simulink model "Controladores_valvula"  (R2014a)
settings: Solver=ode45  StartTime=0.0  StopTime=60  MaxStep=0.1  RelTol=1e-3
values from neighbouring files (symbols this model uses):
  Ap0 = 49.978    [Seccion_5.m]
  Fh0 = 0.8946    [Seccion_5.m]
  Kc_CC_v = 180.7564    [Seccion_5.m]
  Kc_IMC_v = 111.7318    [Seccion_5.m]
  Kc_ZN_v = 155.1600    (= 155.16)    [Seccion_5.m]
  KcPIM_IMC_v = 127.6824    [Seccion_5.m]
  Ki_CC_v = Kc_CC_v/Taoi_CC_v    (= 86.2346262106)    [Seccion_5.m]
  Ki_IMC_v = Kc_IMC_v/Taoi_IMC_v    (= 31.9233714286)    [Seccion_5.m]
  Ki_ZN_v = Kc_ZN_v/Taoi_ZN_v    (= 51.5704457074)    [Seccion_5.m]
  KiPIM_IMC_v = KcPIM_IMC_v/TaoiPIM_IMC_v    (= 31.9237923792)    [Seccion_5.m]
libraries: simulink_need_slupdate x4
settings Model: Creator=lraff  LastModifiedBy=lraff

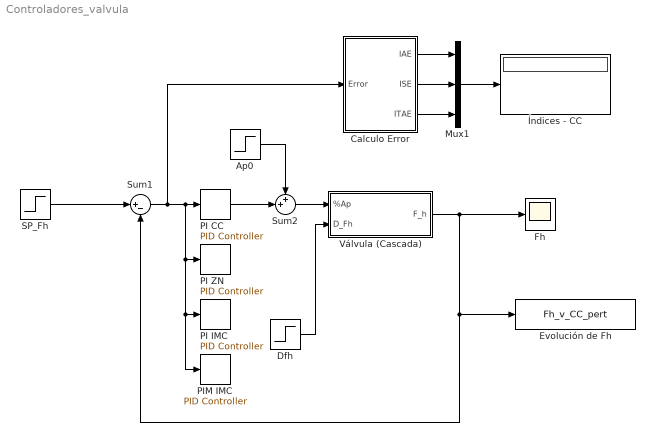
== system Controladores_valvula ==
  Ap0 : Step  Time=0  Before=Ap0  After=Ap0  SampleTime=1
  Calculo Error : Subsystem
  Dfh : Step  Time=10  After=Fh0*0.01  SampleTime=1
  Evolución de Fh : ToWorkspace  VariableName=Fh_v_CC_pert  SaveFormat=Structure With Time
  Fh : Scope
  Mux1 : Mux  Inputs=3
  PI CC : simulink_need_slupdate/PID Controller  P=Kc_CC_v  I=Ki_CC_v  D=0
  PI IMC : simulink_need_slupdate/PID Controller  P=Kc_IMC_v  I=Ki_IMC_v  D=0
  PI ZN : simulink_need_slupdate/PID Controller  P=Kc_ZN_v  I=Ki_ZN_v  D=0
  PIM IMC : simulink_need_slupdate/PID Controller  P=KcPIM_IMC_v  I=KiPIM_IMC_v  D=0
  SP_Fh : Step  Time=10  Before=Fh0  After=Fh0*1  SampleTime=1
  Sum1 : Sum  Inputs=|+-
  Sum2 : Sum  Inputs=++|
  Válvula (Cascada) : Subsystem
  Índices - CC : Display
      settings: SampleTime=1
  wires:
  SP_Fh/1 -> Sum1/1
  Sum1/1 -> PI CC/1, PIM IMC/1, PI IMC/1, PI ZN/1, Calculo Error/1(Error)
  Mux1/1 -> Índices - CC/1
  Calculo Error/1(IAE) -> Mux1/1
  Calculo Error/2(ISE) -> Mux1/2
  Calculo Error/3(ITAE) -> Mux1/3
  Válvula (Cascada)/1(F_h) -> Fh/1, Evolución de Fh/1, Sum1/2
  Ap0/1 -> Sum2/1
  Sum2/1 -> Válvula (Cascada)/1(%Ap)
  PI CC/1 -> Sum2/2
  Dfh/1 -> Válvula (Cascada)/2(D_Fh)

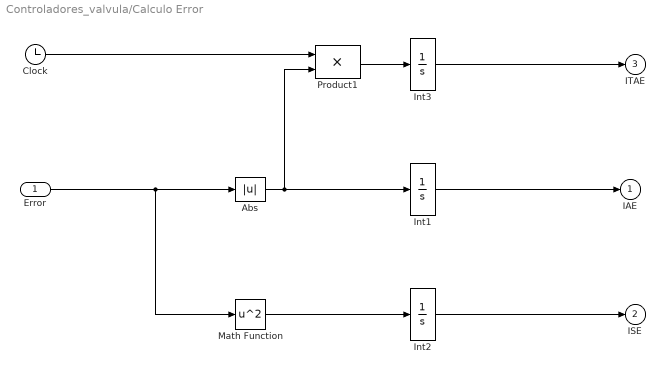
== system Controladores_valvula/Calculo Error ==
  Error : Inport
  Abs : Abs  ZeroCross=off  SaturateOnIntegerOverflow=on
  Clock : Clock
  Int1 : Integrator
  Int2 : Integrator
  Int3 : Integrator
  Math Function : Math  Operator=square  SaturateOnIntegerOverflow=on
  Product1 : Product  SaturateOnIntegerOverflow=on  InputSameDT=on  OutDataTypeStr=Inherit: Same as first input
  IAE : Outport  InitialOutput=0
  ISE : Outport  Port=2  InitialOutput=0
  ITAE : Outport  Port=3  InitialOutput=0
  wires:
  Int1/1 -> IAE/1
  Abs/1 -> Int1/1, Product1/2
  Int2/1 -> ISE/1
  Math Function/1 -> Int2/1
  Clock/1 -> Product1/1
  Product1/1 -> Int3/1
  Int3/1 -> ITAE/1
  Error/1 -> Abs/1, Math Function/1

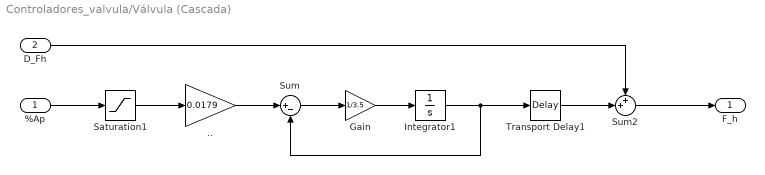
== system Controladores_valvula/Válvula (Cascada) ==
  %Ap : Inport
  D_Fh : Inport  Port=2
  .. : Gain  Gain=0.0179
  Gain : Gain  Gain=1/3.5
  Integrator1 : Integrator  InitialCondition=Fh0
  Saturation1 : Saturate  UpperLimit=100  LowerLimit=0
  Sum : Sum  Inputs=|+-
  Sum2 : Sum  Inputs=++|
  Transport Delay1 : TransportDelay  InitialOutput=Fh0
  F_h : Outport
  wires:
  D_Fh/1 -> Sum2/1
  Sum2/1 -> F_h/1
  %Ap/1 -> Saturation1/1
  Saturation1/1 -> ../1
  Sum/1 -> Gain/1
  Gain/1 -> Integrator1/1
  Integrator1/1 -> Transport Delay1/1, Sum/2
  ../1 -> Sum/1
  Transport Delay1/1 -> Sum2/2
